simulink model "NOLCOlab2Q3"  (R2016b)
settings: Solver=FixedStepAuto  StartTime=0.0  StopTime=20.0  FixedStep=0.001  RelTol=1e-3
settings Model: Creator=akshita_jain  LastModifiedBy=akshita_jain

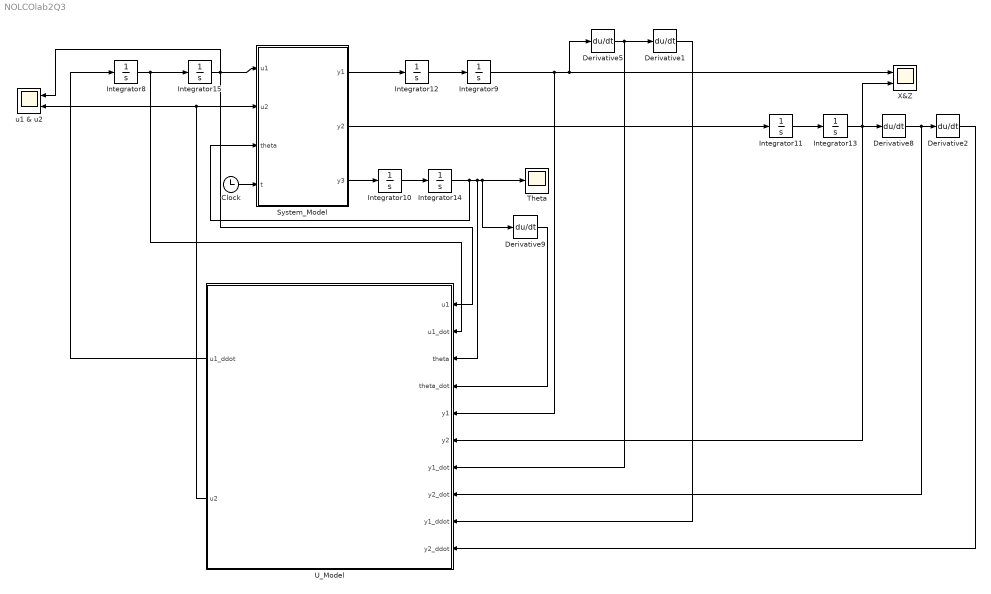
== system NOLCOlab2Q3 ==
  Clock : Clock
  Derivative{1..2,5,8..9} (5 alike) : Derivative
  Integrator{9..10,12,15} (4 alike) : Integrator  InitialCondition=1
  Integrator{8,11,13..14} (4 alike) : Integrator
  System_Model : MATLAB Function  TreatAsAtomicUnit=on
  Theta : Scope
  U_Model : MATLAB Function  TreatAsAtomicUnit=on
  X&Z : Scope  NumInputPorts=2
  u1 & u2 : Scope  NumInputPorts=2
  wires:
  System_Model/2(y2) -> Integrator11/1
  System_Model/3(y3) -> Integrator10/1
  U_Model/1(u1_ddot) -> Integrator8/1
  Integrator9/1 -> X&Z/1, Derivative5/1, U_Model/5(y1)
  Integrator10/1 -> Integrator14/1
  Integrator8/1 -> U_Model/2(u1_dot), Integrator15/1
  Integrator15/1 -> u1 & u2/1, U_Model/1(u1), System_Model/1(u1)
  System_Model/1(y1) -> Integrator12/1
  Integrator12/1 -> Integrator9/1
  Derivative5/1 -> Derivative1/1, U_Model/7(y1_dot)
  Integrator11/1 -> Integrator13/1
  Integrator13/1 -> X&Z/2, Derivative8/1, U_Model/6(y2)
  Derivative8/1 -> Derivative2/1, U_Model/8(y2_dot)
  Derivative9/1 -> U_Model/4(theta_dot)
  Integrator14/1 -> System_Model/3(theta), U_Model/3(theta), Derivative9/1, Theta/1
  Clock/1 -> System_Model/4(t)
  U_Model/2(u2) -> System_Model/2(u2), u1 & u2/2
  Derivative1/1 -> U_Model/9(y1_ddot)
  Derivative2/1 -> U_Model/10(y2_ddot)

== matlab function NOLCOlab2Q3/System_Model ==
  data: u1 input; y1 output; u2 input; theta input; y2 output; y3 output; t input
function [y1,y2,y3] = fcn(u1,u2,theta,t)
delta = 0;
x_ddot = -u1*sin(theta);
z_ddot = u1*cos(theta) - 1;
theta_ddot = u2 + delta * sin(t);

y1 = x_ddot;
y2 = z_ddot;
y3 = theta_ddot;

end

== matlab function NOLCOlab2Q3/U_Model ==
  data: u1 input; u1_dot input; theta input; theta_dot input; u1_ddot output; u2 output; y1 input; y2 input; y1_dot input; y2_dot input; y1_ddot input; y2_ddot input
function [u1_ddot, u2] = fcn(u1,u1_dot,theta,theta_dot,y1,y2,y1_dot,y2_dot,y1_ddot,y2_ddot)
%y1_ddot,y2_dot,y2_ddot,y1_dddot,y2_dddot
%GAINS-
k1 = 400;
k2 = 400;
c1 = 1;
c2 = 3;
c3 = 3;
c4 = 1;

%STATES
y1_dddot = -u1_dot*sin(theta) - u1*theta_dot*cos(theta);
y2_dddot = u1_dot*cos(theta) - u1*theta_dot*sin(theta);

%Sliding Variable
s1 = c1*y1_dddot+c2*y1_ddot+c3*y1_dot+c4*y1;
s2 = c1*y2_dddot+c2*y2_ddot+c3*y2_dot+c4*y2;

%beta matrix
b = [-sin(theta) -u1*cos(theta);cos(theta) -u1*sin(theta)];
%%d = delta*[-u1*cos(theta); -u1*sin(theta)];

%alpha matrix
a1 = -2*u1_dot*cos(theta)*theta_dot + u1*sin(theta)*theta_dot^2+c2*y1_dddot+c3*y1_ddot+c4*y1_dot;
a2 = -2*u1_dot*sin(theta)*theta_dot - u1*cos(theta)*theta_dot^2+c2*y2_dddot+c3*y2_ddot+c4*y2_dot;
a = [a1;a2];

% S variable gain matrix
s_var = [-k1*sign(s1);-k2*sign(s2)];
del = 0.1;
if (abs(s_var) > del)
    sat = sign(s_var);
else
    sat = s_var / del;
end

u = b^-1*(-a + [k1*sat(1);k2*sat(2)]);
u1_ddot = u(1);
u2 = u(2);


end
